simulink model "matprob4"  (R2020b)
settings: Solver=VariableStepAuto  StartTime=0.0  StopTime=10.0  RelTol=1e-3
values from neighbouring files (symbols this model uses):
  b = 3.5077e-06    [matprob4.mat]
  J = 3.2284e-06    [matprob4.mat]
  K = 0.0274    [matprob4.mat]
  L = 2.75e-06    [matprob4.mat]
  R = 4    [matprob4.mat]
settings Model: Creator=Acer  LastModifiedBy=Acer

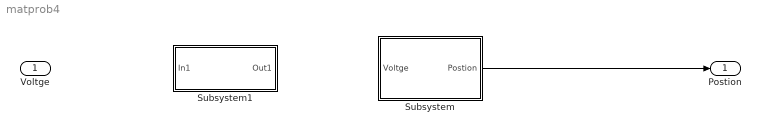
== system matprob4 ==
  Voltge : Inport
  Subsystem : Subsystem
  Subsystem1 : Subsystem
  Postion : Outport
  wires:
  Subsystem/1(Postion) -> Postion/1

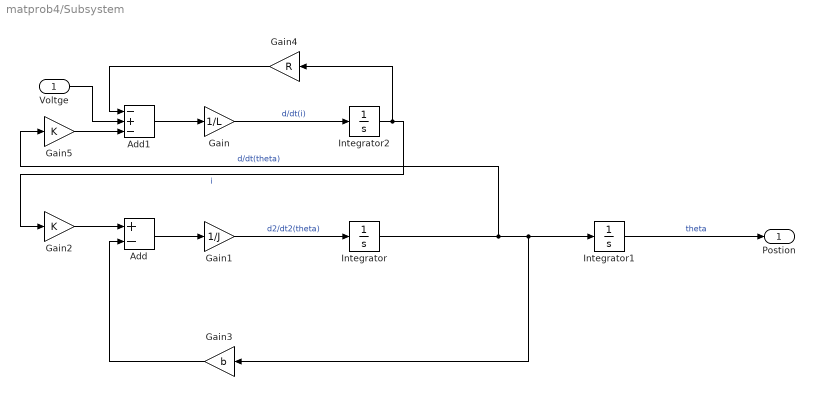
== system matprob4/Subsystem ==
  Voltge : Inport
  Add : Sum  Inputs=+-
  Add1 : Sum  Inputs=-+-
  Gain : Gain  Gain=1/L
  Gain1 : Gain  Gain=1/J
  Gain2 : Gain  Gain=K
  Gain3 : Gain  Gain=b
  Gain4 : Gain  Gain=R
  Gain5 : Gain  Gain=K
  Integrator : Integrator
  Integrator1 : Integrator
  Integrator2 : Integrator
  Postion : Outport
  wires:
  Gain4/1 -> Add1/1
  Gain3/1 -> Add/2
  Gain2/1 -> Add/1
  Gain/1 -> Integrator2/1  "d/dt(i)"
  Integrator2/1 -> Gain4/1, Gain2/1  "i"
  Gain1/1 -> Integrator/1  "d2/dt2(theta)"
  Gain5/1 -> Add1/3
  Add1/1 -> Gain/1
  Integrator1/1 -> Postion/1  "theta"
  Integrator/1 -> Gain5/1, Gain3/1, Integrator1/1  "d/dt(theta)"
  Add/1 -> Gain1/1
  Voltge/1 -> Add1/2

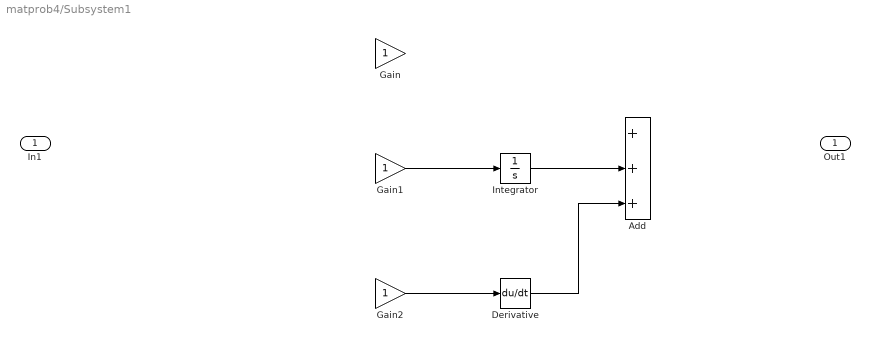
== system matprob4/Subsystem1 ==
  In1 : Inport
  Add : Sum  Inputs=+++
  Derivative : Derivative
  Gain : Gain
  Gain1 : Gain
  Gain2 : Gain
  Integrator : Integrator
  Out1 : Outport
  wires:
  Gain1/1 -> Integrator/1
  Integrator/1 -> Add/2
  Gain2/1 -> Derivative/1
  Derivative/1 -> Add/3
